simulink model "simplified"  (R2019b)
settings: Solver=VariableStepAuto  StartTime=0.0  StopTime=10.0  RelTol=1e-3
model workspace (MAT data in the model file):
  K_b = 1
settings Model: Creator=jasper  LastModifiedBy=jasper

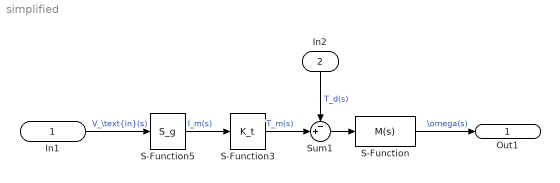
== system simplified ==
  In1 : Inport
  In2 : Inport  Port=2
  S-Function : S-Function  FunctionName=M(s)  SFunctionDeploymentMode=off  EnableBusSupport=off
  S-Function3 : S-Function  FunctionName=K_t  SFunctionDeploymentMode=off  EnableBusSupport=off
  S-Function5 : S-Function  FunctionName=S_g  SFunctionDeploymentMode=off  EnableBusSupport=off
  Sum1 : Sum  Inputs=-+|
  Out1 : Outport
  wires:
  In1/1 -> S-Function5/1  "V_\\text{in}(s)"
  S-Function/1 -> Out1/1  "\\omega(s)"
  S-Function5/1 -> S-Function3/1  "I_m(s)"
  S-Function3/1 -> Sum1/2  "T_m(s)"
  Sum1/1 -> S-Function/1
  In2/1 -> Sum1/1  "T_d(s)"
